simulink model "ProdSys_PennyFab"  (R2015b)
settings: Solver=VariableStepDiscrete  SolverMode=SingleTasking  StartTime=0.0  StopTime=100000  RelTol=1e-3
PostLoadFcn:
  | set_param(gcs, 'Location', [0 0 1750.0, 550.0]);
InitFcn:
  | warning('off','all');
StopFcn:
  | warning('on','all');
libraries: simeventslib x3, simulink x1
Description:
  | % LICENSE:  3-clause "Revised" or "New" or "Modified" BSD License.
  | % Copyright (c) 2015, Georgia Institute of Technology.
  | % All rights reserved.
  | %
  | % Redistribution and use in source and binary forms, with or without
  | % modification, are permitted provided that the following conditions are met:
  | %     * Redistributions of source code must retain the above copyright
  | %       notice, this list of conditions and the following disclaimer.
  | %     * Redistributions in binary form must reproduce the above copyright
  | %       notice, this list of conditions and the following disclaimer in the
  | %       documentation and/or other materials provided with the distribution.
  | %     * Neither the name of the Georgia Institute of Technology nor the
  | %       names of its contributors may be used to endorse or promote products
  | %       derived from this software without specific prior written permission.
  | %
  | % THIS SOFTWARE IS PROVIDED BY THE COPYRIGHT HOLDERS AND CONTRIBUTORS "AS IS" AND
  | % ANY EXPRESS OR IMPLIED WARRANTIES, INCLUDING, BUT NOT LIMITED TO, THE IMPLIED
  | % WARRANTIES OF MERCHANTABILITY AND FITNESS FOR A PARTICULAR PURPOSE ARE
  | % DISCLAIMED. IN NO EVENT SHALL THE GEORGIA INSTITUTE OF TECHNOLOGY BE LIABLE FOR
  | % ANY DIRECT, INDIRECT, INCIDENTAL, SPECIAL, EXEMPLARY, OR CONSEQUENTIAL DAMAGES
  | % (INCLUDING, BUT NOT LIMITED TO, PROCUREMENT OF SUBSTITUTE GOODS OR SERVICES;
  | % LOSS OF USE, DATA, OR PROFITS; OR BUSINESS INTERRUPTION) HOWEVER CAUSED AND
  | % ON ANY THEORY OF LIABILITY, WHETHER IN CONTRACT, STRICT LIABILITY, OR TORT
  | % (INCLUDING NEGLIGENCE OR OTHERWISE) ARISING IN ANY WAY OUT OF THE USE OF THIS
  | % SOFTWARE, EVEN IF ADVISED OF THE POSSIBILITY OF SUCH DAMAGE.
settings Model: Creator=tsprock3  LastModifiedBy=tsprock3
settings DataIOCC: SaveFormat=Array  InspectSignalLogs=on
settings OptimizationCC: BlockReduction=off  BooleanDataType=off
settings DebuggingCC: SaveWithParameterizedLinksMsg=none  UnderspecifiedInitializationDetection=Classic  MergeDetectMultiDrivingBlocksExec=none  SignalResolutionControl=TryResolveAllWithWarning
settings HardwareCC: ProdBitPerPointer=32  ProdLargestAtomicFloat=None  ProdIntDivRoundTo=Undefined  ProdEndianess=Unspecified  ProdWordSize=32  ProdHWDeviceType=32-bit Generic  TargetUnknown=on
settings GRTTargetCC: GeneratePreprocessorConditionals=Disable all
settings ConfigComp: CovModelRefEnable=Off

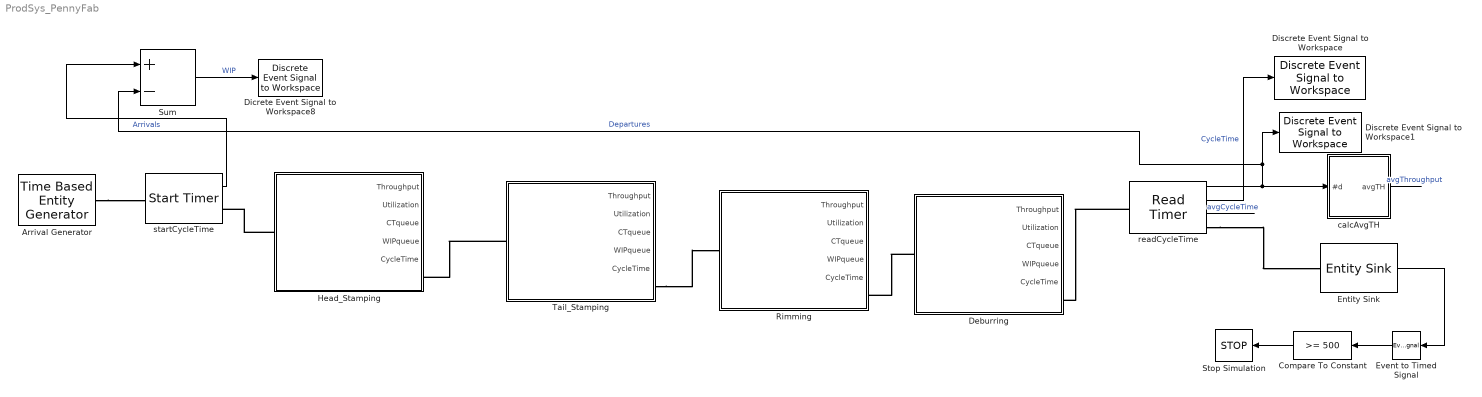
== system ProdSys_PennyFab ==
  Arrival Generator : TimeBasedEntityGenerator  Distribution=Exponential  InitialSeed=46097  Mean=1/.358
  Compare To Constant : simulink/Logic and Bit Operations/Compare To Constant  relop=>=  const=500  OutDataTypeStr=boolean
  Deburring : Subsystem  mask{NumberOfServers=1, Capacity=inf}
      mask prompts: NumberOfServers "m = Number of Parallel Servers"; Capacity "b = buffer size"
      mask TypeOptions NumberOfServers: N-Server/NumberOfServers
      mask TypeOptions Capacity: FIFO Queue/Capacity
  Dicrete Event Signal to Workspace8 : simeventslib/SimEvents Sinks/Discrete Event Signal to Workspace  VariableName=WIP  SaveFormat=Structure With Time  isMonitorOnly=off  isRecordIC=off
  Discrete Event Signal to Workspace : simeventslib/SimEvents Sinks/Discrete Event Signal to Workspace  VariableName=CycleTime  SaveFormat=Structure With Time  isMonitorOnly=off  isRecordIC=off
  Discrete Event Signal to Workspace1 : simeventslib/SimEvents Sinks/Discrete Event Signal to Workspace  VariableName=Departures  SaveFormat=Structure With Time  isMonitorOnly=off  isRecordIC=off
  Entity Sink : EntitySink  StatNumberArrived=on
  Event to Timed Signal : EventToTimedSignal
  Head_Stamping : Subsystem  mask{NumberOfServers=1, Capacity=inf}
      mask prompts: NumberOfServers "m = Number of Parallel Servers"; Capacity "b = buffer size"
      mask TypeOptions NumberOfServers: N-Server/NumberOfServers
      mask TypeOptions Capacity: FIFO Queue/Capacity
  Rimming : Subsystem  mask{NumberOfServers=1, Capacity=inf}
      mask prompts: NumberOfServers "m = Number of Parallel Servers"; Capacity "b = buffer size"
      mask TypeOptions NumberOfServers: N-Server/NumberOfServers
      mask TypeOptions Capacity: FIFO Queue/Capacity
  Stop Simulation : Stop
  Sum : Sum  Inputs=|+-
  Tail_Stamping : Subsystem  mask{NumberOfServers=1, Capacity=inf}
      mask prompts: NumberOfServers "m = Number of Parallel Servers"; Capacity "b = buffer size"
      mask TypeOptions NumberOfServers: N-Server/NumberOfServers
      mask TypeOptions Capacity: FIFO Queue/Capacity
  calcAvgTH : Subsystem
  readCycleTime : ReadTimer  TimerTag=CycleTime  StatNumberDeparted=on  StatTimeElapsed=on  StatAverageTimeElapsed=on
      settings: OutputPortMap=o0,o2,o3
  startCycleTime : StartTimer  TimerTag=CycleTime  TimerStartedOption=Restart  StatNumberDeparted=on
  wires:
  readCycleTime/2 -> Discrete Event Signal to Workspace/1  "CycleTime"
  Sum/1 -> Dicrete Event Signal to Workspace8/1  "WIP"
  startCycleTime/1 -> Sum/1  "Arrivals"
  readCycleTime/1 -> Sum/2, Discrete Event Signal to Workspace1/1, calcAvgTH/1(#d)  "Departures"
  readCycleTime/3 -> ?  "avgCycleTime"
  calcAvgTH/1(avgTH) -> ?  "avgThroughput"
  Entity Sink/1 -> Event to Timed Signal/1
  Compare To Constant/1 -> Stop Simulation/1
  Event to Timed Signal/1 -> Compare To Constant/1
  connections:
  readCycleTime/RConn1 -- Entity Sink/LConn1
  Head_Stamping/LConn1 -- startCycleTime/RConn1
  Arrival Generator/RConn1 -- startCycleTime/LConn1
  readCycleTime/LConn1 -- Deburring/RConn1
  Tail_Stamping/RConn1 -- Rimming/LConn1
  Deburring/LConn1 -- Rimming/RConn1
  Tail_Stamping/LConn1 -- Head_Stamping/RConn1

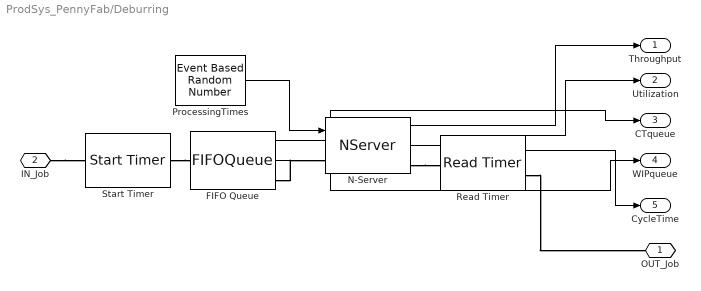
== system ProdSys_PennyFab/Deburring ==
  FIFO Queue : FIFOQueue  Capacity=Capacity  StatAverageWait=on  StatAverageQueueLength=on
      settings: OutputPortMap=o2,o3
  N-Server : NServer  NumberOfServers=NumberOfServers  ServiceTimeFrom=Signal port t  StatNumberDeparted=on  StatUtilization=on
      settings: OutputPortMap=o0,o5
  ProcessingTimes : EventBasedRandomNumber  meanExp=2  meanNorm=5  stdNorm=2  Seed=1
  Read Timer : ReadTimer  TimerTag=WorkstationCycleTime  StatAverageTimeElapsed=on
      settings: OutputPortMap=o3
  Start Timer : StartTimer  TimerTag=WorkstationCycleTime  TimerStartedOption=Restart
  OUT_Job : PMIOPort  Port=1  Side=Right
  IN_Job : PMIOPort  Port=2  Side=Left
  Throughput : Outport
  Utilization : Outport  Port=2
  CTqueue : Outport  Port=3
  WIPqueue : Outport  Port=4
  CycleTime : Outport  Port=5
  wires:
  ProcessingTimes/1 -> N-Server/1
  N-Server/1 -> Throughput/1
  N-Server/2 -> Utilization/1
  FIFO Queue/1 -> CTqueue/1
  FIFO Queue/2 -> WIPqueue/1
  Read Timer/1 -> CycleTime/1
  connections:
  FIFO Queue/RConn1 -- N-Server/LConn1
  IN_Job/RConn1 -- Start Timer/LConn1
  Start Timer/RConn1 -- FIFO Queue/LConn1
  N-Server/RConn1 -- Read Timer/LConn1
  Read Timer/RConn1 -- OUT_Job/RConn1

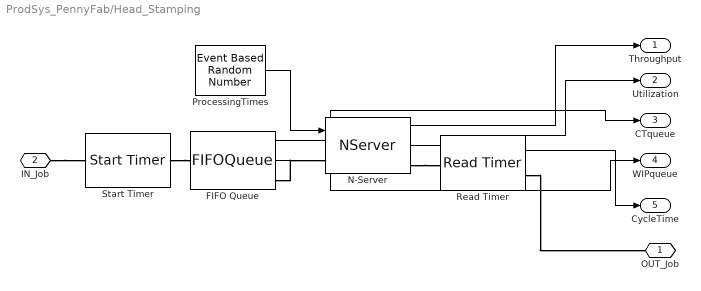
== system ProdSys_PennyFab/Head_Stamping ==
  FIFO Queue : FIFOQueue  Capacity=Capacity  StatAverageWait=on  StatAverageQueueLength=on
      settings: OutputPortMap=o2,o3
  N-Server : NServer  NumberOfServers=NumberOfServers  ServiceTimeFrom=Signal port t  StatNumberDeparted=on  StatUtilization=on
      settings: OutputPortMap=o0,o5
  ProcessingTimes : EventBasedRandomNumber  meanExp=2  meanNorm=5  stdNorm=2  Seed=1
  Read Timer : ReadTimer  TimerTag=WorkstationCycleTime  StatAverageTimeElapsed=on
      settings: OutputPortMap=o3
  Start Timer : StartTimer  TimerTag=WorkstationCycleTime  TimerStartedOption=Restart
  OUT_Job : PMIOPort  Port=1  Side=Right
  IN_Job : PMIOPort  Port=2  Side=Left
  Throughput : Outport
  Utilization : Outport  Port=2
  CTqueue : Outport  Port=3
  WIPqueue : Outport  Port=4
  CycleTime : Outport  Port=5
  wires:
  ProcessingTimes/1 -> N-Server/1
  N-Server/1 -> Throughput/1
  N-Server/2 -> Utilization/1
  FIFO Queue/1 -> CTqueue/1
  FIFO Queue/2 -> WIPqueue/1
  Read Timer/1 -> CycleTime/1
  connections:
  FIFO Queue/RConn1 -- N-Server/LConn1
  IN_Job/RConn1 -- Start Timer/LConn1
  Start Timer/RConn1 -- FIFO Queue/LConn1
  N-Server/RConn1 -- Read Timer/LConn1
  Read Timer/RConn1 -- OUT_Job/RConn1

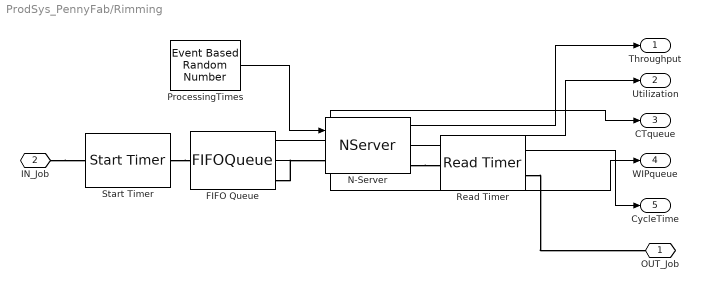
== system ProdSys_PennyFab/Rimming ==
  FIFO Queue : FIFOQueue  Capacity=Capacity  StatAverageWait=on  StatAverageQueueLength=on
      settings: OutputPortMap=o2,o3
  N-Server : NServer  NumberOfServers=NumberOfServers  ServiceTimeFrom=Signal port t  StatNumberDeparted=on  StatUtilization=on
      settings: OutputPortMap=o0,o5
  ProcessingTimes : EventBasedRandomNumber  meanExp=2  meanNorm=5  stdNorm=2  Seed=1
  Read Timer : ReadTimer  TimerTag=WorkstationCycleTime  StatAverageTimeElapsed=on
      settings: OutputPortMap=o3
  Start Timer : StartTimer  TimerTag=WorkstationCycleTime  TimerStartedOption=Restart
  OUT_Job : PMIOPort  Port=1  Side=Right
  IN_Job : PMIOPort  Port=2  Side=Left
  Throughput : Outport
  Utilization : Outport  Port=2
  CTqueue : Outport  Port=3
  WIPqueue : Outport  Port=4
  CycleTime : Outport  Port=5
  wires:
  ProcessingTimes/1 -> N-Server/1
  N-Server/1 -> Throughput/1
  N-Server/2 -> Utilization/1
  FIFO Queue/1 -> CTqueue/1
  FIFO Queue/2 -> WIPqueue/1
  Read Timer/1 -> CycleTime/1
  connections:
  FIFO Queue/RConn1 -- N-Server/LConn1
  IN_Job/RConn1 -- Start Timer/LConn1
  Start Timer/RConn1 -- FIFO Queue/LConn1
  N-Server/RConn1 -- Read Timer/LConn1
  Read Timer/RConn1 -- OUT_Job/RConn1

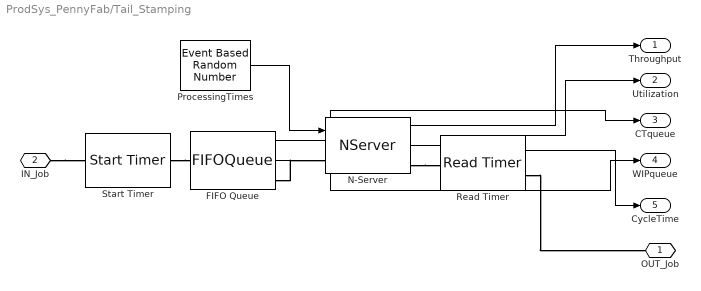
== system ProdSys_PennyFab/Tail_Stamping ==
  FIFO Queue : FIFOQueue  Capacity=Capacity  StatAverageWait=on  StatAverageQueueLength=on
      settings: OutputPortMap=o2,o3
  N-Server : NServer  NumberOfServers=NumberOfServers  ServiceTimeFrom=Signal port t  StatNumberDeparted=on  StatUtilization=on
      settings: OutputPortMap=o0,o5
  ProcessingTimes : EventBasedRandomNumber  meanExp=2  meanNorm=5  stdNorm=2  Seed=1
  Read Timer : ReadTimer  TimerTag=WorkstationCycleTime  StatAverageTimeElapsed=on
      settings: OutputPortMap=o3
  Start Timer : StartTimer  TimerTag=WorkstationCycleTime  TimerStartedOption=Restart
  OUT_Job : PMIOPort  Port=1  Side=Right
  IN_Job : PMIOPort  Port=2  Side=Left
  Throughput : Outport
  Utilization : Outport  Port=2
  CTqueue : Outport  Port=3
  WIPqueue : Outport  Port=4
  CycleTime : Outport  Port=5
  wires:
  ProcessingTimes/1 -> N-Server/1
  N-Server/1 -> Throughput/1
  N-Server/2 -> Utilization/1
  FIFO Queue/1 -> CTqueue/1
  FIFO Queue/2 -> WIPqueue/1
  Read Timer/1 -> CycleTime/1
  connections:
  FIFO Queue/RConn1 -- N-Server/LConn1
  IN_Job/RConn1 -- Start Timer/LConn1
  Start Timer/RConn1 -- FIFO Queue/LConn1
  N-Server/RConn1 -- Read Timer/LConn1
  Read Timer/RConn1 -- OUT_Job/RConn1

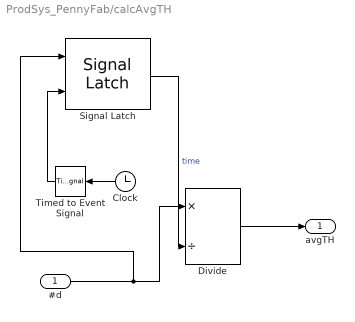
== system ProdSys_PennyFab/calcAvgTH ==
  #d : Inport
  Clock : Clock
  Divide : Product  Inputs=*/
  Signal Latch : SignalLatch  ReadMemoryUpon=Write to memory event
      settings: InputPortMap=u0,u2  OutputPortMap=o2
  Timed to Event Signal : TimedToEventSignal
  avgTH : Outport
  wires:
  #d/1 -> Signal Latch/1, Divide/1
  Timed to Event Signal/1 -> Signal Latch/2
  Signal Latch/1 -> Divide/2  "time"
  Clock/1 -> Timed to Event Signal/1
  Divide/1 -> avgTH/1
